simulink library "constantSetpoints_cl"  (R2018b)
settings: Solver=VariableStepAuto  StartTime=0.0  StopTime=10.0  RelTol=1e-3
libraries: filteredPDController_ul x3, slrtlib x2
settings Model: Creator=mcobb  LastModifiedBy=mae-ncsucore

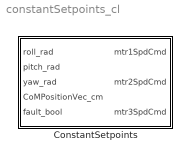
== system constantSetpoints_cl ==
  ConstantSetpoints : Subsystem

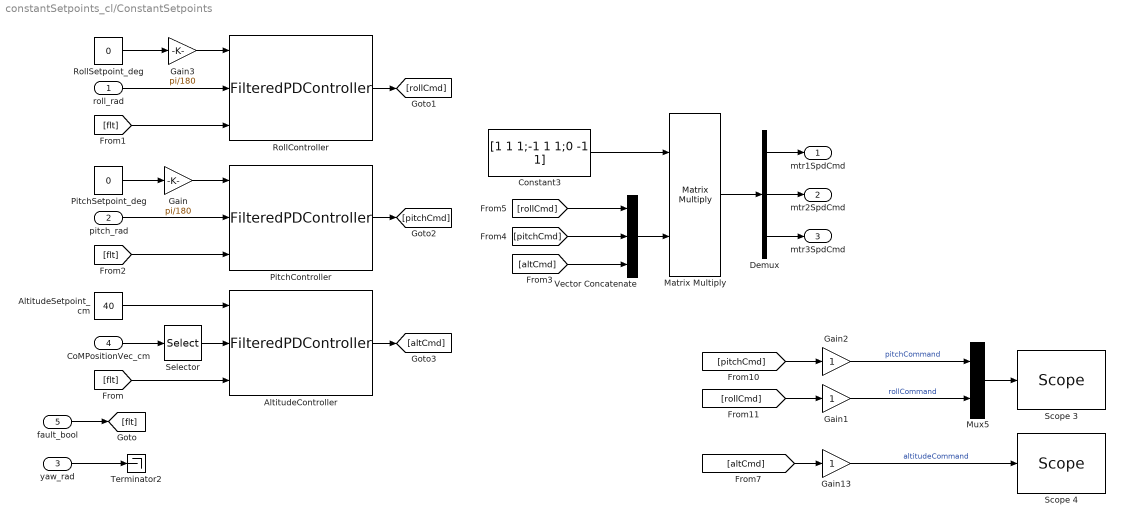
== system constantSetpoints_cl/ConstantSetpoints ==
  roll_rad : Inport
  pitch_rad : Inport  Port=2
  yaw_rad : Inport  Port=3
  CoMPositionVec_cm : Inport  Port=4
  fault_bool : Inport  Port=5  OutDataTypeStr=boolean
  AltitudeController : filteredPDController_ul/FilteredPDController  enable=on  kp=1  kd=0  timeConstant_s=0.1  intialError=0  initialOutput=0
  AltitudeSetpoint_cm : Constant  Value=40
  Constant3 : Constant  Value=[1 1 1;-1 1 1;0 -1 1]
  Demux : Demux  Outputs=3
  Gain : Gain  Gain=pi/180
  Gain1 : Gain
  Gain13 : Gain
  Gain2 : Gain
  Gain3 : Gain  Gain=pi/180
  Matrix Multiply : Product  Multiplication=Matrix(*)
  Mux5 : Mux  Inputs=2
  PitchController : filteredPDController_ul/FilteredPDController  enable=on  kp=1  kd=0  timeConstant_s=0.1  intialError=0  initialOutput=0
  PitchSetpoint_deg : Constant  Value=0
  RollController : filteredPDController_ul/FilteredPDController  enable=on  kp=1  kd=0  timeConstant_s=0.1  intialError=0  initialOutput=0
  RollSetpoint_deg : Constant  Value=0
  Scope 3 : slrtlib/Displays and Logging/Scope   scopeno=2  scopetype=Target  autostart=on  viewmode=Graphical rolling  formatstr='%15.6f'  grid=on  ylimits=[-1.5,1.5]  nosamples=1000  noprepostsamples=0  interleave=1  triggermode=FreeRun  triggersignal=1  trigsignalfromport=off  triggerlevel=0.0  triggerslope=Either  triggerscope=1  triggersample=0  filename=data.dat  mode=Lazy  writesize=512  autorestart=off  dynamicfilemode=off  maxwritefilesize=512*1024^2
  Scope 4 : slrtlib/Displays and Logging/Scope   scopeno=4  scopetype=Target  autostart=on  viewmode=Graphical rolling  formatstr='%15.6f'  grid=on  ylimits=[0,0]  nosamples=1000  noprepostsamples=0  interleave=1  triggermode=FreeRun  triggersignal=1  trigsignalfromport=off  triggerlevel=0.0  triggerslope=Either  triggerscope=1  triggersample=0  filename=data.dat  mode=Lazy  writesize=512  autorestart=off  dynamicfilemode=off  maxwritefilesize=512*1024^2
  Selector : Selector  InputPortWidth=3  IndexOptions=Index vector (dialog)  Indices=3  OutputSizes=1
  Terminator2 : Terminator
  Vector Concatenate : Concatenate  NumInputs=3
  mtr1SpdCmd : Outport
  mtr2SpdCmd : Outport  Port=2
  mtr3SpdCmd : Outport  Port=3
  wires:
  roll_rad/1 -> RollController/2
  pitch_rad/1 -> PitchController/2
  yaw_rad/1 -> Terminator2/1
  CoMPositionVec_cm/1 -> Selector/1
  RollSetpoint_deg/1 -> Gain3/1
  PitchSetpoint_deg/1 -> Gain/1
  AltitudeSetpoint_cm/1 -> AltitudeController/1
  [rollCmd] -> Vector Concatenate/1
  Vector Concatenate/1 -> Matrix Multiply/2
  Constant3/1 -> Matrix Multiply/1
  [pitchCmd] -> Vector Concatenate/2
  [altCmd] -> Vector Concatenate/3
  Demux/1 -> mtr1SpdCmd/1
  Demux/2 -> mtr2SpdCmd/1
  Demux/3 -> mtr3SpdCmd/1
  Matrix Multiply/1 -> Demux/1
  Selector/1 -> AltitudeController/2
  fault_bool/1 -> [flt]
  [flt] -> AltitudeController/3
  [flt] -> RollController/3
  [flt] -> PitchController/3
  AltitudeController/1 -> [altCmd]
  [rollCmd] -> Gain1/1
  [pitchCmd] -> Gain2/1
  Mux5/1 -> Scope 3/1
  [altCmd] -> Gain13/1
  Gain13/1 -> Scope 4/1  "altitudeCommand"
  Gain1/1 -> Mux5/2  "rollCommand"
  Gain2/1 -> Mux5/1  "pitchCommand"
  Gain/1 -> PitchController/1
  Gain3/1 -> RollController/1
  RollController/1 -> [rollCmd]
  PitchController/1 -> [pitchCmd]
